simulink model "ThreeSinglePhaseDiodeRectifierWithoutLSchematic_2"  (R2018a)
settings: Solver=VariableStepAuto  StartTime=0.0  StopTime=1  RelTol=1e-3
libraries: powerlib x17, powerlib_meascontrol x1
settings Model: Creator=mertelmas  LastModifiedBy=mertelmas

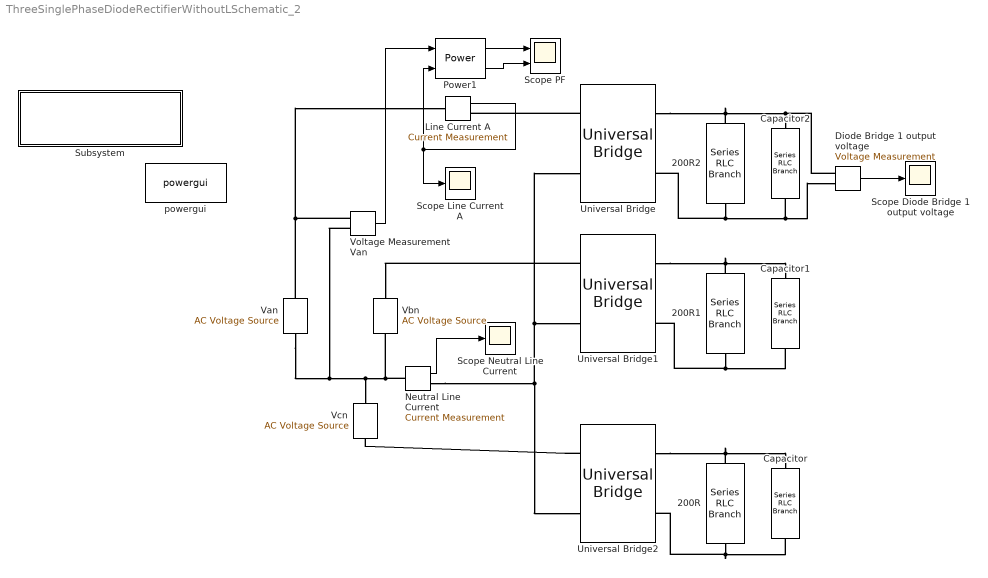
== system ThreeSinglePhaseDiodeRectifierWithoutLSchematic_2 ==
  200R : powerlib/Elements/Series RLC Branch  LConnTagsString=__new0  RConnTagsString=__new0  BranchType=R  Resistance=200  Inductance=1e-3  SetiL0=off  InitialCurrent=0  Capacitance=1e-6  Setx0=off  InitialVoltage=0  Measurements=None
  200R1 : powerlib/Elements/Series RLC Branch  LConnTagsString=__new0  RConnTagsString=__new0  BranchType=R  Resistance=200  Inductance=1e-3  SetiL0=off  InitialCurrent=0  Capacitance=1e-6  Setx0=off  InitialVoltage=0  Measurements=None
  200R2 : powerlib/Elements/Series RLC Branch  LConnTagsString=__new0  RConnTagsString=__new0  BranchType=R  Resistance=200  Inductance=1e-3  SetiL0=off  InitialCurrent=0  Capacitance=1e-6  Setx0=off  InitialVoltage=0  Measurements=None
  Capacitor : powerlib/Elements/Series RLC Branch  LConnTagsString=__new0  RConnTagsString=__new0  BranchType=C  Resistance=1  Inductance=1e-3  SetiL0=off  InitialCurrent=0  Capacitance=47e-5  Setx0=off  InitialVoltage=0  Measurements=None
  Capacitor1 : powerlib/Elements/Series RLC Branch  LConnTagsString=__new0  RConnTagsString=__new0  BranchType=C  Resistance=1  Inductance=1e-3  SetiL0=off  InitialCurrent=0  Capacitance=47e-5  Setx0=off  InitialVoltage=0  Measurements=None
  Capacitor2 : powerlib/Elements/Series RLC Branch  LConnTagsString=__new0  RConnTagsString=__new0  BranchType=C  Resistance=1  Inductance=1e-3  SetiL0=off  InitialCurrent=0  Capacitance=47e-5  Setx0=off  InitialVoltage=0  Measurements=None
  Diode Bridge 1 output voltage : powerlib/Measurements/Voltage Measurement  PhasorSimulation=off  OutputType=Complex  PSBequivalent=0
  Line Current A : powerlib/Measurements/Current Measurement  PhasorSimulation=off  OutputType=Complex  PSBequivalent=0
  Neutral Line Current : powerlib/Measurements/Current Measurement  PhasorSimulation=off  OutputType=Complex  PSBequivalent=0
  Power1 : powerlib_meascontrol/Measurements/Power  Freq=50  Vinit=[1, 0]  Iinit=[1, 0]  Ts=0
      settings: SourceProductName=Simscape Power Systems
  Scope Line Current A : Scope
  Scope Neutral Line Current : Scope
  Scope Diode Bridge 1 output voltage : Scope
  Scope PF : Scope  NumInputPorts=2
  Subsystem : Subsystem
      settings: OpenFcn=open_system('power_new_palette')
      mask Display: disp(sprintf('Open Simscape Power Systems\n(Specialized Technology)\nPalette Library'));
  Universal Bridge : powerlib/Power Electronics/Universal Bridge  Arms=2  SnubberResistance=1e5  SnubberCapacitance=inf  Device=Diodes  Ron=1e-3  Lon=0  ForwardVoltages="[  0  0  ]"  ForwardVoltage=0  GTOparameters=[ 10e-6 , 20e-6 ]  IGBTparameters=[ 1e-6 , 2e-6 ]  Measurements=None  Measurements_2=None  converterType=Rectifier
  Universal Bridge1 : powerlib/Power Electronics/Universal Bridge  Arms=2  SnubberResistance=1e5  SnubberCapacitance=inf  Device=Diodes  Ron=1e-3  Lon=0  ForwardVoltages="[  0  0  ]"  ForwardVoltage=0  GTOparameters=[ 10e-6 , 20e-6 ]  IGBTparameters=[ 1e-6 , 2e-6 ]  Measurements=None  Measurements_2=None  converterType=Rectifier
  Universal Bridge2 : powerlib/Power Electronics/Universal Bridge  Arms=2  SnubberResistance=1e5  SnubberCapacitance=inf  Device=Diodes  Ron=1e-3  Lon=0  ForwardVoltages="[  0  0  ]"  ForwardVoltage=0  GTOparameters=[ 10e-6 , 20e-6 ]  IGBTparameters=[ 1e-6 , 2e-6 ]  Measurements=None  Measurements_2=None  converterType=Rectifier
  Van : powerlib/Electrical Sources/AC Voltage Source  Amplitude=325.27  Phase=0  Frequency=50  SampleTime=0  Measurements=None  BusType=swing  Pref=10e3  Qref=0  Qmin=-inf  Qmax=+inf
  Vbn : powerlib/Electrical Sources/AC Voltage Source  Amplitude=325.27  Phase=120  Frequency=50  SampleTime=0  Measurements=None  BusType=swing  Pref=10e3  Qref=0  Qmin=-inf  Qmax=+inf
  Vcn : powerlib/Electrical Sources/AC Voltage Source  Amplitude=325.27  Phase=240  Frequency=50  SampleTime=0  Measurements=None  BusType=swing  Pref=10e3  Qref=0  Qmin=-inf  Qmax=+inf
  Voltage Measurement Van : powerlib/Measurements/Voltage Measurement  PhasorSimulation=off  OutputType=Complex  PSBequivalent=0
  powergui : powerlib/powergui  Priority=1  SimulationMode=Discrete  SampleTime=10e-6  frequency=60  Iterations=50  frequencyindice=50  Pbase=100e6  ErrMax=1e-4  UnitsV=kV  UnitsW=MW  buscounter=0  FunctionMessages=off  echomessages=off  EnableUseOfTLC=off  CurrentSourceSwitches=off  DisableSnubberDevices=off  DisableRonSwitches=off  DisableVfSwitches=off  DisplayEquations=off  SolverType=Tustin/Backward Euler (TBE)  Interpol=off  ExternalGateDelay=off  methode=off  Ts=100  x0status=blocks  SPID=off  SwTol=0  HookPort=off  RestoreLinks=warning  ResistiveCurrentMeasurement=off  Frange=[0:2:500]  Ylog=off  Xlog=on  ShowGrid=off  save=off  variable=ZData  structure=LineCurrentAWithoutL  ZoomFFT=off  StartTime=0.2  cycles=10  DisplayStyle=1  fundamental=50  FreqAxis=off  MaxFrequency=1000  frequencyindicesteady=1  RmsSteady=2  display=off
  wires:
  Neutral Line Current/1 -> Scope Neutral Line Current/1
  Diode Bridge 1 output voltage/1 -> Scope Diode Bridge 1 output voltage/1
  Voltage Measurement Van/1 -> Power1/1
  Line Current A/1 -> Power1/2, Scope Line Current A/1
  Power1/2 -> Scope PF/2
  Power1/1 -> Scope PF/1
  connections:
  Universal Bridge2/RConn1 -- 200R/LConn1 -- Capacitor/LConn1
  Capacitor2/RConn1 -- Diode Bridge 1 output voltage/LConn2 -- 200R2/RConn1 -- Universal Bridge/RConn2
  Diode Bridge 1 output voltage/LConn1 -- Universal Bridge/RConn1 -- 200R2/LConn1 -- Capacitor2/LConn1
  Neutral Line Current/RConn1 -- Universal Bridge2/LConn2 -- Universal Bridge/LConn2 -- Universal Bridge1/LConn2
  Universal Bridge1/RConn1 -- 200R1/LConn1 -- Capacitor1/LConn1
  Van/LConn1 -- Voltage Measurement Van/LConn2 -- Neutral Line Current/LConn1 -- Vbn/LConn1 -- Vcn/LConn1
  200R/RConn1 -- Capacitor/RConn1 -- Universal Bridge2/RConn2
  Universal Bridge1/RConn2 -- 200R1/RConn1 -- Capacitor1/RConn1
  Van/RConn1 -- Voltage Measurement Van/LConn1 -- Line Current A/LConn1
  Universal Bridge/LConn1 -- Line Current A/RConn1
  Universal Bridge1/LConn1 -- Vbn/RConn1
  Universal Bridge2/LConn1 -- Vcn/RConn1

== system ThreeSinglePhaseDiodeRectifierWithoutLSchematic_2/Subsystem ==
